simulink model "ModelThrusters"  (R2022b)
settings: Solver=VariableStepAuto  StartTime=0.0  StopTime=20  RelTol=1e-3
values from neighbouring files (symbols this model uses):
  Roll_thrust_operator = abs(-1/( (1/(norm(Params.arm_vec1)))*(-sin(gamma1)*cos(theta)*Params.arm_vec1(3)+cos(gamma1)*Params.arm_vec1(2))+         (1/(norm(Params.arm_vec2)))*(-sin(gamma2)*cos(theta)*Params.arm_vec2(3)+cos(gamma2)*Params.arm_vec2(2))+         (1/(norm(Params.arm_vec3)))*(sin(gamma3)*sin(theta)*Params.arm_vec3(3)-cos(gamma3)*Params.arm_vec3(1))+         (1/(norm(Params.arm_vec4)))*(sin(gamma4)*cos(theta)*P ...(+51 chars)    [Detumbling_using_engine_SimCode.m]
  tau_Thrusters = 30e-03    (= 0.03)    [Detumbling_using_engine_SimCode.m]
undefined symbols (not defined in the file or in its folder): Params, Roll, T1, time_T2, time_T3, time_T4
libraries: matrix_library x4
settings Model: Creator=שקד  LastModifiedBy=שקד
settings SolverCC: AlgebraicLoopSolver=TrustRegion
settings DebuggingCC: UnconnectedInputMsg=warning  UnconnectedOutputMsg=warning  UnconnectedLineMsg=warning  SFMachineParentedDataDiag=warning
settings ModelReferenceCC: EnableRefExpFcnMdlSchedulingChecks=on

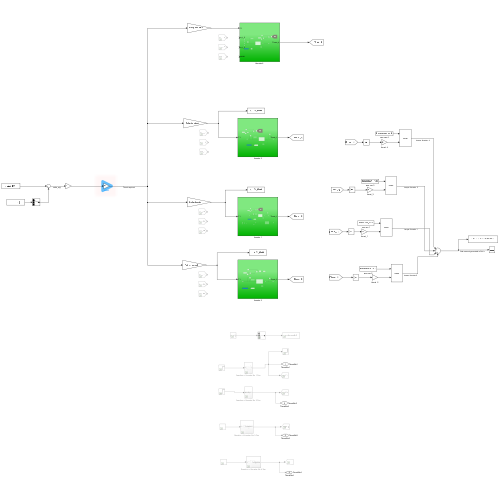
[thumbnail: Simulink's stored preview of the top-level diagram]
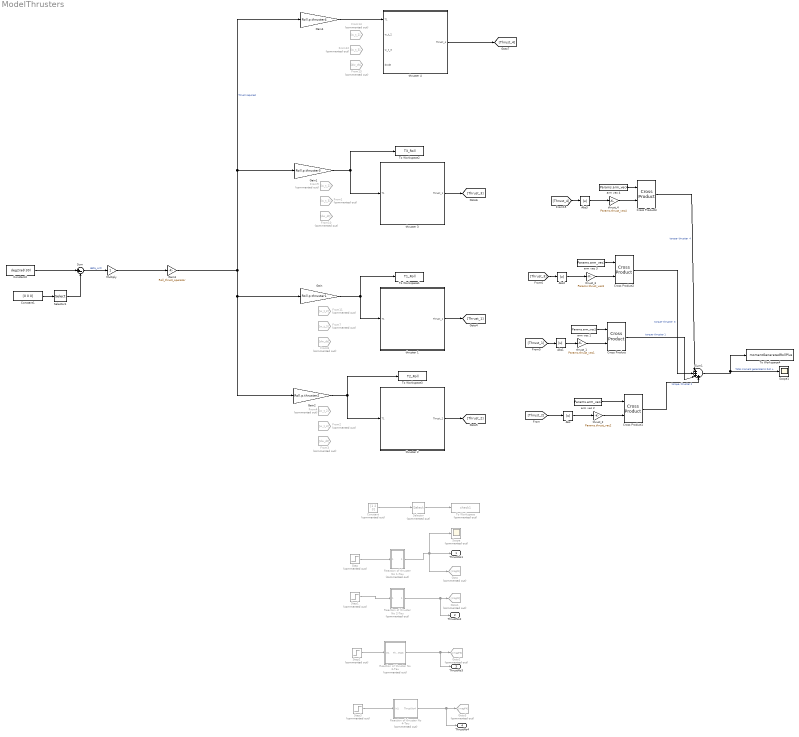
== system ModelThrusters ==
  Abs{,1..3} (4 alike) : Abs  SaturateOnIntegerOverflow=off
  Constant : Constant  Commented=on  Value=[1 2 3]
  Constant1 : Constant  Value=[0 0 0]
  Constant2 : Constant  Value=deg2rad(30)
  Cross Product{,1..3} (4 alike) : matrix_library/Cross Product
  From{1..2,7,12} (4 alike) : From  Commented=on  GotoTag=w_t_3
  From{3,8,10,13} (4 alike) : From  Commented=on  GotoTag=dw_dt
  From{4,9,11,14} (4 alike) : From  Commented=on  GotoTag=w_t_2
  Gain : Gain  Gain=Roll.p.thruster1
  Gain1 : Gain  Gain=Roll.p.thruster3
  Gain2 : Gain  Gain=Roll.p.thruster2
  Gain3 : Gain  Gain=Roll_thrust_operator
  Gain4 : Gain  Gain=Roll.p.thruster4
  Goto : Goto  Commented=on  GotoTag=magF1
  Goto1 : Goto  Commented=on  GotoTag=magF2
  Goto2 : Goto  Commented=on  GotoTag=magF3
  Goto3 : Goto  Commented=on  GotoTag=magF4
  Multiply : Gain
  "Reaction of thruster No 1-Tau " : Subsystem  Commented=on
  "Reaction of thruster No 2-Tau " : Subsystem  Commented=on
  "Reaction of thruster No 3-Tau " : Subsystem  Commented=on
  "Reaction of thruster No 4-Tau " : Subsystem  Commented=on
  Scope : Scope  Commented=on
  Scope1 : Scope
  Selector : Selector  Commented=on  InputPortWidth=3  IndexOptions=Index vector (dialog)  Indices=[2]  OutputSizes=1
  Selector1 : Selector  InputPortWidth=3  IndexOptions=Index vector (dialog)  Indices=[1]  OutputSizes=1
  Step : Step  Commented=on  Time=50  Before=7  After=7  SampleTime=0
  Step1 : Step  Commented=on  Time=0  Before=1  SampleTime=0
  Step2 : Step  Commented=on  Time=0  Before=1  SampleTime=0
  Step3 : Step  Commented=on  Time=0  Before=1  SampleTime=0
  Sum : Sum  Inputs=|+-
  Sum1 : Sum  Inputs=|++++
  To Workspace : ToWorkspace  Commented=on  VariableName=check1  SaveFormat=Timeseries  SampleTime=-1
  To Workspace1 : ToWorkspace  VariableName=T1_Roll  SaveFormat=Timeseries  SampleTime=-1
  To Workspace2 : ToWorkspace  VariableName=T3_Roll  SaveFormat=Timeseries  SampleTime=-1
  To Workspace3 : ToWorkspace  VariableName=T2_Roll  SaveFormat=Timeseries  SampleTime=-1
  To Workspace4 : ToWorkspace  VariableName=momentGeneratedRollPlus  SaveFormat=Timeseries  SampleTime=-1
  arm vec 1 : Constant  Value=Params.arm_vec1
  arm vec 2 : Constant  Value=Params.arm_vec2
  arm vec 3 : Constant  Value=Params.arm_vec3
  arm vec 4 : Constant  Value=Params.arm_vec4
  thrust_1 : Gain  Gain=Params.thrust_vec1
  thrust_2 : Gain  Gain=Params.thrust_vec2
  thrust_3 : Gain  Gain=Params.thrust_vec3
  thrust_4 : Gain  Gain=Params.thrust_vec4
  thruster 1 : Subsystem
  thruster 2 : Subsystem
  thruster 3 : Subsystem
  "thruster 4 " : Subsystem
  ThrustNo1 : Outport  SignalName=ThrustNo1  SampleTime=0.01
  ThrustNo2 : Outport  Port=2  SignalName=ThrustNo2  SampleTime=0.01
  ThrustNo3 : Outport  Port=3  SignalName=ThrustNo3  SampleTime=0.01
  ThrustNo4 : Outport  Port=4  SignalName=ThrustNo4  SampleTime=0.01
  wires:
  Step/1 -> "Reaction of thruster No 1-Tau "/1(In1)
  Step1/1 -> "Reaction of thruster No 2-Tau "/1(In1)
  Step2/1 -> "Reaction of thruster No 3-Tau "/1(In1)
  Step3/1 -> "Reaction of thruster No 4-Tau "/1(In1)
  "Reaction of thruster No 2-Tau "/1(ThrustNo2) -> ThrustNo2/1, Goto1/1
  "Reaction of thruster No 3-Tau "/1(ThrustNo3) -> ThrustNo3/1, Goto2/1
  "Reaction of thruster No 4-Tau "/1(ThrustNo4) -> ThrustNo4/1, Goto3/1
  "Reaction of thruster No 1-Tau "/1(Out1) -> ThrustNo1/1, Goto/1, Scope/1
  Constant/1 -> Selector/1
  Selector/1 -> To Workspace/1
  thruster 1/1(Thrust_1) -> [Thrust_1]
  thruster 2/1(Thrust_2) -> [Thrust_2]
  thrust_1/1 -> Cross Product/2
  Sum1/1 -> To Workspace4/1, Scope1/1  "Total moment generated in Roll +"
  Abs/1 -> thrust_2/1
  [Thrust_1] -> Abs1/1
  Cross Product/1 -> Sum1/3  "torque- thruster 1"
  [Thrust_2] -> Abs/1
  Abs1/1 -> thrust_1/1
  thrust_2/1 -> Cross Product1/2
  Cross Product1/1 -> Sum1/4  "torque- thruster 2"
  arm vec 2/1 -> Cross Product1/1
  arm vec 1/1 -> Cross Product/1
  Constant1/1 -> Selector1/1
  Sum/1 -> Multiply/1  "delta_w(t)"
  Constant2/1 -> Sum/1
  Selector1/1 -> Sum/2
  Abs2/1 -> thrust_3/1
  Cross Product2/1 -> Sum1/2  "torque- thruster  3"
  arm vec 3/1 -> Cross Product2/1
  thrust_3/1 -> Cross Product2/2
  thruster 3/1(Thrust_1) -> [Thrust_3]
  [Thrust_3] -> Abs2/1
  Gain/1 -> To Workspace1/1, thruster 1/1(T1)
  Gain1/1 -> To Workspace2/1, thruster 3/1(T1)
  Gain2/1 -> To Workspace3/1, thruster 2/1(T1)
  Multiply/1 -> Gain3/1
  Gain3/1 -> Gain2/1, Gain/1, Gain4/1, Gain1/1  "Thrust required"
  "thruster 4 "/1(Thrust_4) -> [Thrust_4]
  Gain4/1 -> "thruster 4 "/1(T1)
  Cross Product3/1 -> Sum1/1  "torque- thruster  4"
  Abs3/1 -> thrust_4/1
  thrust_4/1 -> Cross Product3/2
  arm vec 4/1 -> Cross Product3/1
  [Thrust_4] -> Abs3/1

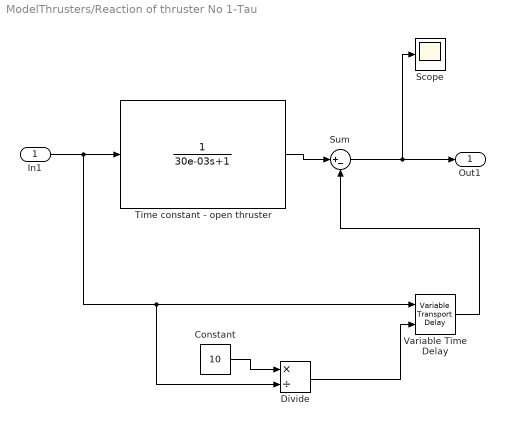
== system ModelThrusters/Reaction of thruster No 1-Tau  ==
  In1 : Inport
  Constant : Constant  Value=10
  Divide : Product  Inputs=*/
  Scope : Scope
  Sum : Sum  Inputs=|+-
  "Time constant - open thruster " : TransferFcn  Denominator=[30e-03 1]
  Variable Time Delay : VariableTransportDelay  MaximumDelay=30
  Out1 : Outport
  wires:
  Sum/1 -> Scope/1, Out1/1
  "Time constant - open thruster "/1 -> Sum/1
  In1/1 -> Divide/2, Variable Time Delay/1, "Time constant - open thruster "/1
  Variable Time Delay/1 -> Sum/2
  Divide/1 -> Variable Time Delay/2
  Constant/1 -> Divide/1

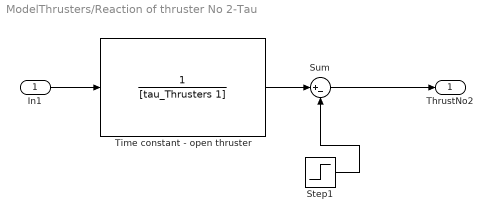
== system ModelThrusters/Reaction of thruster No 2-Tau  ==
  In1 : Inport
  Step1 : Step  Time=time_T2  SampleTime=0
  Sum : Sum  Inputs=|+-
  "Time constant - open thruster " : TransferFcn  Denominator=[tau_Thrusters 1]
  ThrustNo2 : Outport
  wires:
  Sum/1 -> ThrustNo2/1
  Step1/1 -> Sum/2
  "Time constant - open thruster "/1 -> Sum/1
  In1/1 -> "Time constant - open thruster "/1

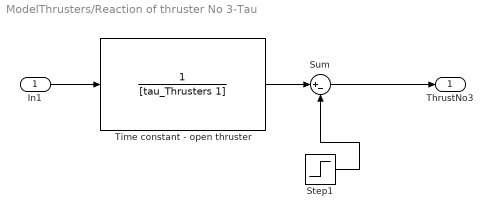
== system ModelThrusters/Reaction of thruster No 3-Tau  ==
  In1 : Inport
  Step1 : Step  Time=time_T3  SampleTime=0
  Sum : Sum  Inputs=|+-
  "Time constant - open thruster " : TransferFcn  Denominator=[tau_Thrusters 1]
  ThrustNo3 : Outport
  wires:
  Sum/1 -> ThrustNo3/1
  Step1/1 -> Sum/2
  "Time constant - open thruster "/1 -> Sum/1
  In1/1 -> "Time constant - open thruster "/1

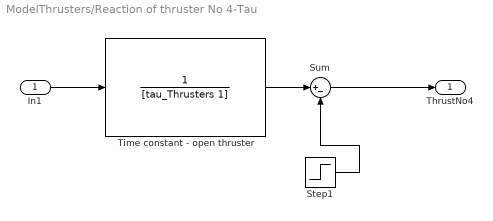
== system ModelThrusters/Reaction of thruster No 4-Tau  ==
  In1 : Inport
  Step1 : Step  Time=time_T4  SampleTime=0
  Sum : Sum  Inputs=|+-
  "Time constant - open thruster " : TransferFcn  Denominator=[tau_Thrusters 1]
  ThrustNo4 : Outport
  wires:
  Sum/1 -> ThrustNo4/1
  Step1/1 -> Sum/2
  "Time constant - open thruster "/1 -> Sum/1
  In1/1 -> "Time constant - open thruster "/1

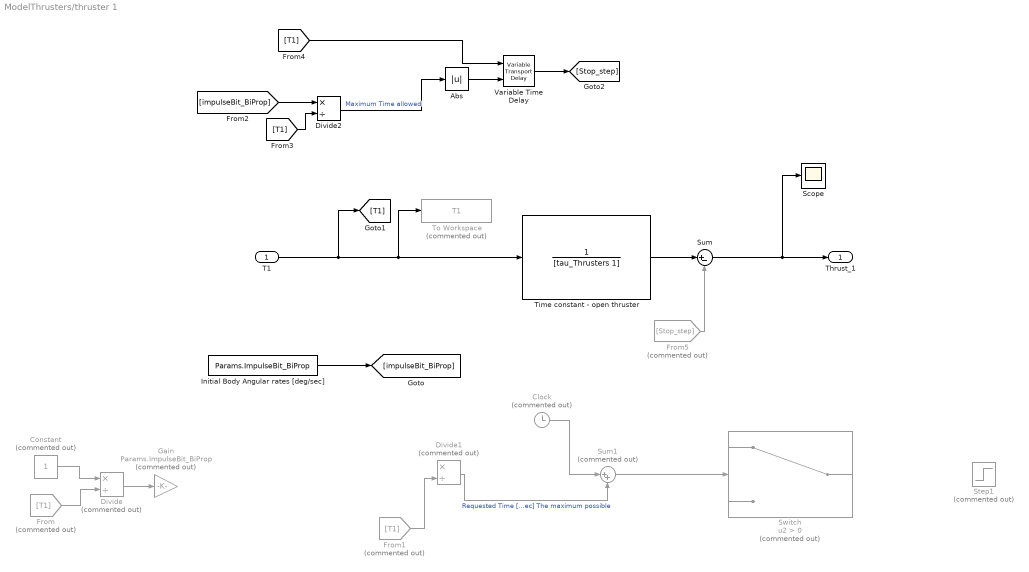
== system ModelThrusters/thruster 1 ==
  T1 : Inport
  Abs : Abs  SaturateOnIntegerOverflow=off
  Clock : Clock  Commented=on
  Constant : Constant  Commented=on
  Divide : Product  Commented=on  Inputs=*/
  Divide1 : Product  Commented=on  Inputs=*/
  Divide2 : Product  Inputs=*/
  From : From  Commented=on  GotoTag=T1
  From1 : From  Commented=on  GotoTag=T1
  From5 : From  Commented=on  GotoTag=Stop_step
  Gain : Gain  Commented=on  Gain=Params.ImpulseBit_BiProp
  Initial Body Angular rates [deg/sec] : Constant  Value=Params.ImpulseBit_BiProp
  Scope : Scope
  Step1 : Step  Commented=on  Time=Params.ImpulseBit_BiProp/T1  SampleTime=0
  Sum : Sum  Inputs=|+-
  Sum1 : Sum  Commented=on  Inputs=|++
  Switch : Switch  Commented=on  Criteria=u2 > Threshold  SaturateOnIntegerOverflow=off  InputSameDT=off
  "Time constant - open thruster " : TransferFcn  Denominator=[tau_Thrusters 1]
  To Workspace : ToWorkspace  Commented=on  VariableName=T1  SaveFormat=Timeseries  SampleTime=-1
  Variable Time Delay : VariableTransportDelay  MaximumDelay=50
  Thrust_1 : Outport
  wires:
  "Time constant - open thruster "/1 -> Sum/1
  Sum/1 -> Scope/1, Thrust_1/1
  Initial Body Angular rates [deg/sec]/1 -> [impulseBit_BiProp]
  Constant/1 -> Divide/1
  From/1 -> Divide/2
  Divide/1 -> Gain/1
  From1/1 -> Divide1/2
  Divide1/1 -> Sum1/2  "Requested Time [sec] The maximum possible"
  Clock/1 -> Sum1/1
  Sum1/1 -> Switch/2
  T1/1 -> [T1], To Workspace/1, "Time constant - open thruster "/1
  Divide2/1 -> Abs/1  "Maximum Time allowed"
  [impulseBit_BiProp] -> Divide2/1
  [T1] -> Divide2/2
  [T1] -> Variable Time Delay/1
  Variable Time Delay/1 -> [Stop_step]
  From5/1 -> Sum/2
  Abs/1 -> Variable Time Delay/2

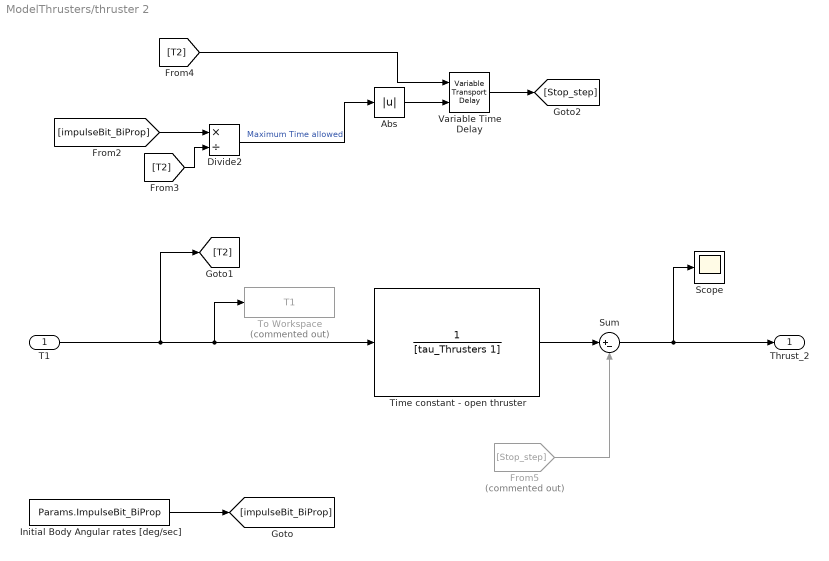
== system ModelThrusters/thruster 2 ==
  T1 : Inport
  Abs : Abs  SaturateOnIntegerOverflow=off
  Divide2 : Product  Inputs=*/
  From5 : From  Commented=on  GotoTag=Stop_step
  Initial Body Angular rates [deg/sec] : Constant  Value=Params.ImpulseBit_BiProp
  Scope : Scope
  Sum : Sum  Inputs=|+-
  "Time constant - open thruster " : TransferFcn  Denominator=[tau_Thrusters 1]
  To Workspace : ToWorkspace  Commented=on  VariableName=T1  SaveFormat=Timeseries  SampleTime=-1
  Variable Time Delay : VariableTransportDelay  MaximumDelay=50
  Thrust_2 : Outport
  wires:
  "Time constant - open thruster "/1 -> Sum/1
  Sum/1 -> Scope/1, Thrust_2/1
  Initial Body Angular rates [deg/sec]/1 -> [impulseBit_BiProp]
  T1/1 -> [T2], To Workspace/1, "Time constant - open thruster "/1
  [T2] -> Divide2/2
  Divide2/1 -> Abs/1  "Maximum Time allowed"
  [T2] -> Variable Time Delay/1
  Variable Time Delay/1 -> [Stop_step]
  [impulseBit_BiProp] -> Divide2/1
  From5/1 -> Sum/2
  Abs/1 -> Variable Time Delay/2

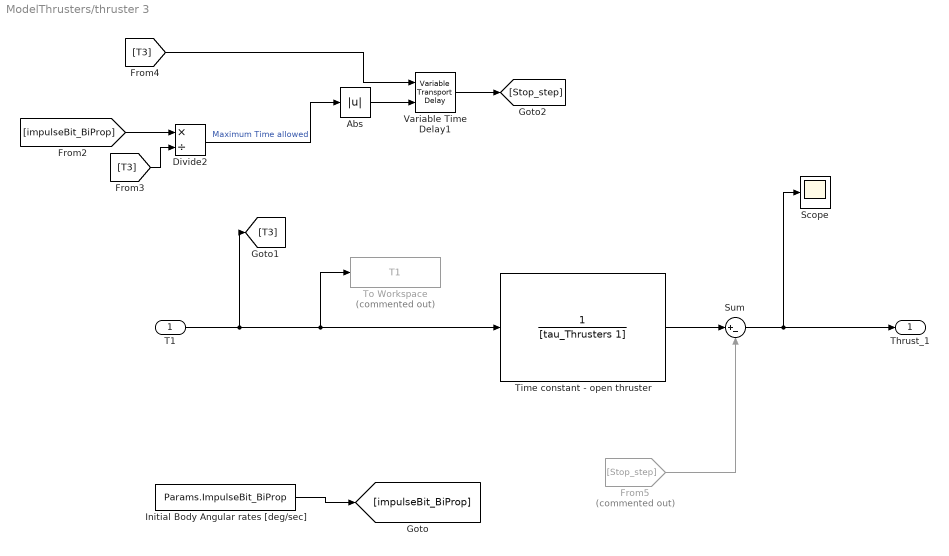
== system ModelThrusters/thruster 3 ==
  T1 : Inport
  Abs : Abs  SaturateOnIntegerOverflow=off
  Divide2 : Product  Inputs=*/
  From5 : From  Commented=on  GotoTag=Stop_step
  Initial Body Angular rates [deg/sec] : Constant  Value=Params.ImpulseBit_BiProp
  Scope : Scope
  Sum : Sum  Inputs=|+-
  "Time constant - open thruster " : TransferFcn  Denominator=[tau_Thrusters 1]
  To Workspace : ToWorkspace  Commented=on  VariableName=T1  SaveFormat=Timeseries  SampleTime=-1
  Variable Time Delay1 : VariableTransportDelay  MaximumDelay=50
  Thrust_1 : Outport
  wires:
  "Time constant - open thruster "/1 -> Sum/1
  Sum/1 -> Scope/1, Thrust_1/1
  Initial Body Angular rates [deg/sec]/1 -> [impulseBit_BiProp]
  T1/1 -> [T3], To Workspace/1, "Time constant - open thruster "/1
  [T3] -> Divide2/2
  Divide2/1 -> Abs/1  "Maximum Time allowed"
  [T3] -> Variable Time Delay1/1
  Variable Time Delay1/1 -> [Stop_step]
  [impulseBit_BiProp] -> Divide2/1
  From5/1 -> Sum/2
  Abs/1 -> Variable Time Delay1/2

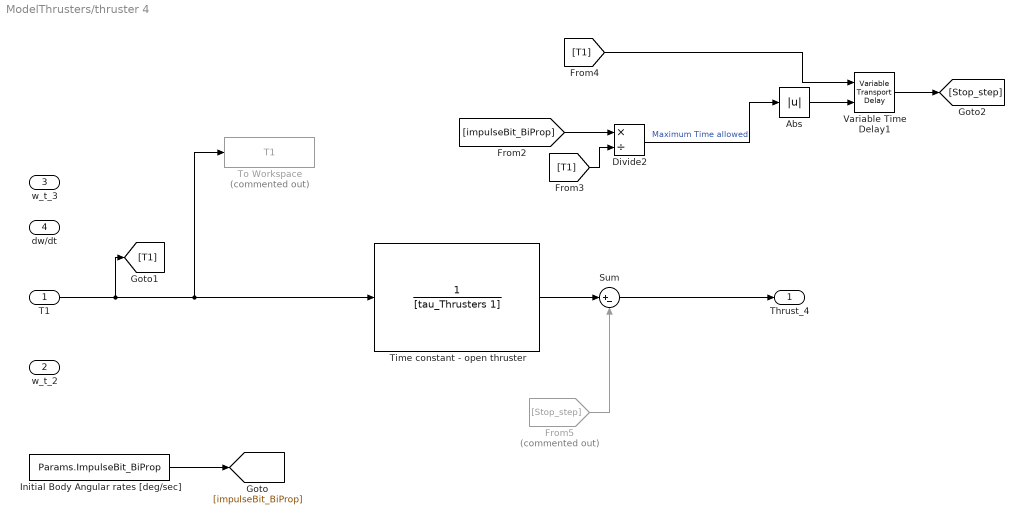
== system ModelThrusters/thruster 4  ==
  T1 : Inport
  w_t_2 : Inport  Port=2
  w_t_3 : Inport  Port=3
  dw/dt : Inport  Port=4
  Abs : Abs  SaturateOnIntegerOverflow=off
  Divide2 : Product  Inputs=*/
  From5 : From  Commented=on  GotoTag=Stop_step
  Initial Body Angular rates [deg/sec] : Constant  Value=Params.ImpulseBit_BiProp
  Sum : Sum  Inputs=|+-
  "Time constant - open thruster " : TransferFcn  Denominator=[tau_Thrusters 1]
  To Workspace : ToWorkspace  Commented=on  VariableName=T1  SaveFormat=Timeseries  SampleTime=-1
  Variable Time Delay1 : VariableTransportDelay  MaximumDelay=50
  Thrust_4 : Outport
  wires:
  "Time constant - open thruster "/1 -> Sum/1
  Sum/1 -> Thrust_4/1
  Initial Body Angular rates [deg/sec]/1 -> [impulseBit_BiProp]
  T1/1 -> [T1], To Workspace/1, "Time constant - open thruster "/1
  [impulseBit_BiProp] -> Divide2/1
  [T1] -> Divide2/2
  Divide2/1 -> Abs/1  "Maximum Time allowed"
  [T1] -> Variable Time Delay1/1
  Variable Time Delay1/1 -> [Stop_step]
  From5/1 -> Sum/2
  Abs/1 -> Variable Time Delay1/2
